simulink model "vtg_r24b"  (R2024b)
settings: Solver=FixedStepAuto  StartTime=0.0  StopTime=inf  FixedStep=0.05  RelTol=1e-3
libraries: robotlib x13
settings Model: Creator=sprinkle  LastModifiedBy=Shaimaa ElBaklish
settings OptimizationCC: DefaultParameterBehavior=Inlined  EnhancedBackFolding=on  PassReuseOutputArgsAs=Individual arguments  ZeroExternalMemoryAtStartup=off  ZeroInternalMemoryAtStartup=off  MaxStackSize=64  OptimizeBlockOrder=speed  DifferentSizesBufferReuse=on  OptimizationCustomize=off  EfficientTunableParamExpr=on
settings DebuggingCC: ParameterTunabilityLossMsg=error
settings HardwareCC: ProdBitPerPointer=32  ProdBitPerSizeT=32  ProdBitPerPtrDiffT=32  ProdLargestAtomicFloat=None  ProdIntDivRoundTo=Undefined  ProdEndianess=Unspecified  ProdWordSize=32  ProdHWDeviceType=Generic->Unspecified (assume 32-bit Generic)
settings SFSimCC: MATLABDynamicMemAlloc=off
settings RTWCC: Description=Embedded Coder  SystemTargetFile=ert.tlc  HardwareBoard=Robot Operating System (ROS)  TLCOptions="-aInlineSetEventsForThisBaseRateFcn=TLC_FALSE -aSuppressMultiTaskScheduler=TLC_FALSE  -aRateBasedStepFcn=0"  GenCodeOnly=on  TemplateMakefile=ert_default_tmf  Toolchain=Catkin  TargetLang=C++
settings CodeAppCC: ForceParamTrailComments=on  IgnoreCustomStorageClasses=off  OperatorAnnotations=on  SimulinkDataObjDesc=on  SFDataObjDesc=on  InsertBlockDesc=on

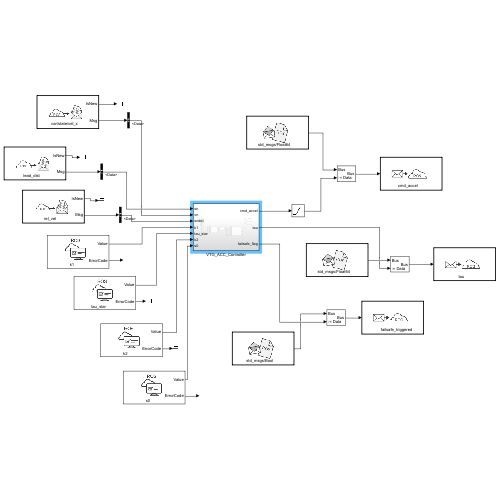
[thumbnail: Simulink's stored preview of the top-level diagram]
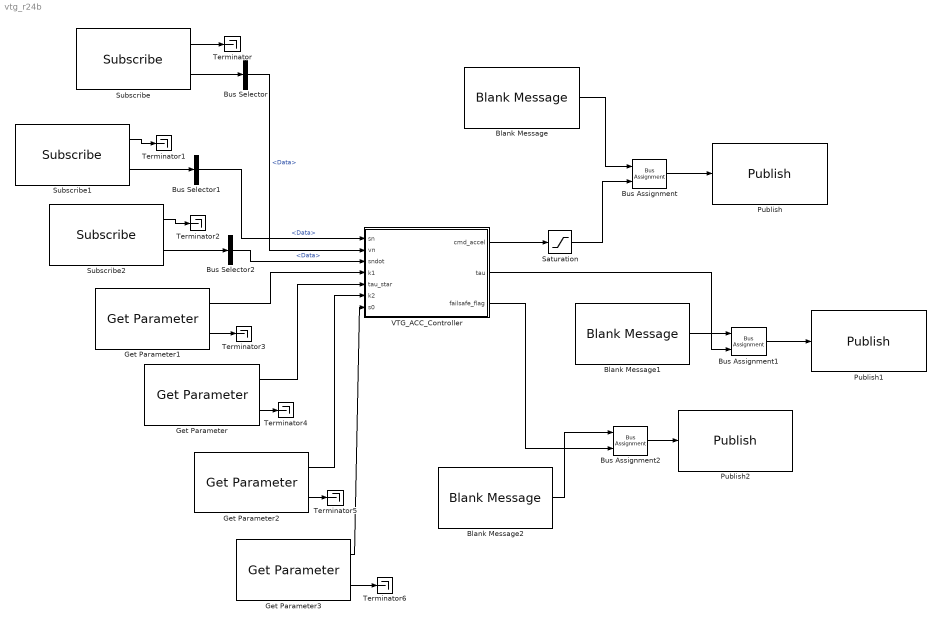
== system vtg_r24b ==
  Blank Message : robotlib/Blank Message  messageClass=Message  entityType=std_msgs/Float64  messageType=std_msgs/Float64  SampleTime=inf  legacyBusStruct=off
  Blank Message1 : robotlib/Blank Message  messageClass=Message  entityType=std_msgs/Float64  messageType=std_msgs/Float64  SampleTime=inf  legacyBusStruct=off
  Blank Message2 : robotlib/Blank Message  messageClass=Message  entityType=std_msgs/Bool  messageType=std_msgs/Bool  SampleTime=inf  legacyBusStruct=off
  Bus Assignment : BusAssignment  AssignedSignals=Data
  Bus Assignment1 : BusAssignment  AssignedSignals=Data
  Bus Assignment2 : BusAssignment  AssignedSignals=Data
  Bus Selector : BusSelector  OutputSignals=Data
  Bus Selector1 : BusSelector  OutputSignals=Data
  Bus Selector2 : BusSelector  OutputSignals=Data
  Get Parameter : robotlib/Get Parameter  ParameterSource=Specify your own  ParameterName=tau_star  ParameterType=double  ParameterMaxArrayLength=16  ParameterInitialValue=2.0  SampleTime=-1  ShowErrorCodeOutput=on  ModelName=vtg_r24b  BlockId=ParamGet_vtg_r24b_18
  Get Parameter1 : robotlib/Get Parameter  ParameterSource=Specify your own  ParameterName=k1  ParameterType=double  ParameterMaxArrayLength=16  ParameterInitialValue=1.1  SampleTime=-1  ShowErrorCodeOutput=on  ModelName=vtg_r24b  BlockId=ParamGet_vtg_r24b_19
  Get Parameter2 : robotlib/Get Parameter  ParameterSource=Specify your own  ParameterName=k2  ParameterType=double  ParameterMaxArrayLength=16  ParameterInitialValue=0.1  SampleTime=-1  ShowErrorCodeOutput=on  ModelName=vtg_r24b  BlockId=ParamGet_vtg_r24b_52
  Get Parameter3 : robotlib/Get Parameter  ParameterSource=Specify your own  ParameterName=s0  ParameterType=double  ParameterMaxArrayLength=16  ParameterInitialValue=0.1  SampleTime=-1  ShowErrorCodeOutput=on  ModelName=vtg_r24b  BlockId=ParamGet_vtg_r24b_54
  Publish : robotlib/Publish  topicSource=Specify your own  topic=cmd_accel  messageType=std_msgs/Float64  legacyBusStruct=off  messageQueueLength=1
  Publish1 : robotlib/Publish  topicSource=Specify your own  topic=tau  messageType=std_msgs/Float64  legacyBusStruct=off  messageQueueLength=1
  Publish2 : robotlib/Publish  topicSource=Specify your own  topic=failsafe_triggered  messageType=std_msgs/Float64  legacyBusStruct=off  messageQueueLength=1
  Saturation : Saturate  UpperLimit=1.5  LowerLimit=-3.0
  Subscribe : robotlib/Subscribe  topicSource=Specify your own  topic=car/state/vel_x  messageType=std_msgs/Float64  SampleTime=-1  legacyBusStruct=off  messageQueueLength=1
  Subscribe1 : robotlib/Subscribe  topicSource=Specify your own  topic=lead_dist  messageType=std_msgs/Float64  SampleTime=-1  legacyBusStruct=off  messageQueueLength=1
  Subscribe2 : robotlib/Subscribe  topicSource=Specify your own  topic=rel_vel  messageType=std_msgs/Float64  SampleTime=-1  legacyBusStruct=off  messageQueueLength=1
  Terminator{,1..6} (7 alike) : Terminator
  VTG_ACC_Controller : Subsystem
  wires:
  Subscribe/2 -> Bus Selector/1
  Subscribe/1 -> Terminator/1
  Subscribe1/1 -> Terminator1/1
  Blank Message/1 -> Bus Assignment/1
  Bus Assignment/1 -> Publish/1
  Bus Selector/1 -> VTG_ACC_Controller/2(vn)  "<Data>"
  VTG_ACC_Controller/1(cmd_accel) -> Saturation/1
  Get Parameter/1 -> VTG_ACC_Controller/5(tau_star)
  Get Parameter1/1 -> VTG_ACC_Controller/4(k1)
  Saturation/1 -> Bus Assignment/2
  Subscribe1/2 -> Bus Selector1/1
  Bus Selector1/1 -> VTG_ACC_Controller/1(sn)  "<Data>"
  Subscribe2/1 -> Terminator2/1
  Bus Selector2/1 -> VTG_ACC_Controller/3(sndot)  "<Data>"
  Subscribe2/2 -> Bus Selector2/1
  Get Parameter1/2 -> Terminator3/1
  Get Parameter/2 -> Terminator4/1
  Get Parameter2/1 -> VTG_ACC_Controller/6(k2)
  Get Parameter2/2 -> Terminator5/1
  Get Parameter3/2 -> Terminator6/1
  Get Parameter3/1 -> VTG_ACC_Controller/7(s0)
  Bus Assignment1/1 -> Publish1/1
  VTG_ACC_Controller/2(tau) -> Bus Assignment1/2
  Blank Message1/1 -> Bus Assignment1/1
  VTG_ACC_Controller/3(failsafe_flag) -> Bus Assignment2/2
  Blank Message2/1 -> Bus Assignment2/1
  Bus Assignment2/1 -> Publish2/1

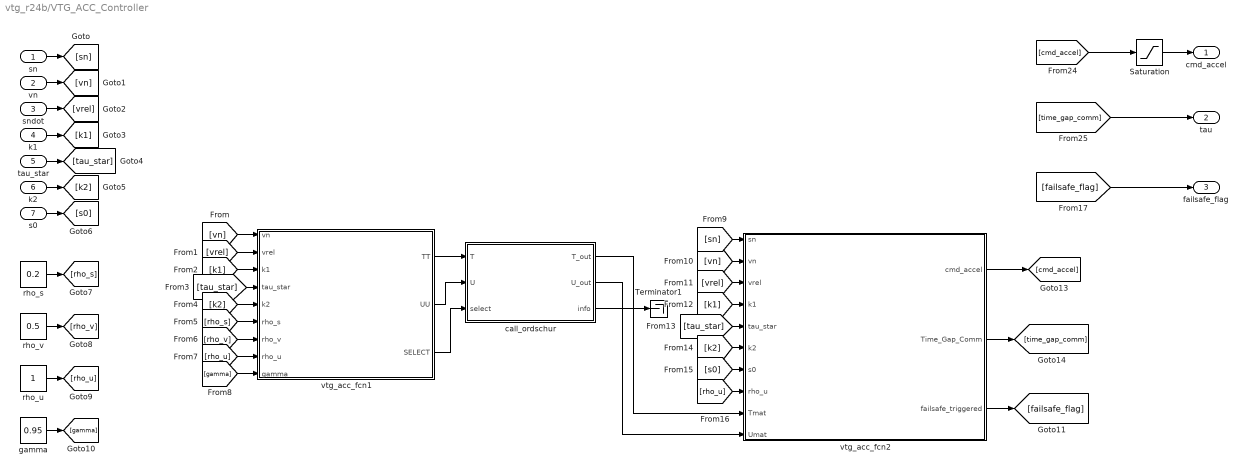
== system vtg_r24b/VTG_ACC_Controller ==
  sn : Inport
  vn : Inport  Port=2
  sndot : Inport  Port=3
  k1 : Inport  Port=4
  tau_star : Inport  Port=5
  k2 : Inport  Port=6
  s0 : Inport  Port=7
  Saturation : Saturate  UpperLimit=1.5  LowerLimit=-3
  Terminator1 : Terminator
  call_ordschur : MATLAB Function  TreatAsAtomicUnit=on
  gamma : Constant  Value=0.95
  rho_s : Constant  Value=0.2
  rho_u : Constant
  rho_v : Constant  Value=0.5
  vtg_acc_fcn1 : MATLAB Function  TreatAsAtomicUnit=on
  vtg_acc_fcn2 : MATLAB Function  TreatAsAtomicUnit=on
  cmd_accel : Outport
  tau : Outport  Port=2
  failsafe_flag : Outport  Port=3
  wires:
  Saturation/1 -> cmd_accel/1
  vtg_acc_fcn1/1(TT) -> call_ordschur/1(T)
  vtg_acc_fcn1/2(UU) -> call_ordschur/2(U)
  vtg_acc_fcn1/3(SELECT) -> call_ordschur/3(select)
  call_ordschur/1(T_out) -> vtg_acc_fcn2/9(Tmat)
  call_ordschur/3(info) -> Terminator1/1
  sn/1 -> [sn]
  vn/1 -> [vn]
  sndot/1 -> [vrel]
  k1/1 -> [k1]
  tau_star/1 -> [tau_star]
  k2/1 -> [k2]
  s0/1 -> [s0]
  rho_s/1 -> [rho_s]
  rho_v/1 -> [rho_v]
  rho_u/1 -> [rho_u]
  gamma/1 -> [gamma]
  [vn] -> vtg_acc_fcn1/1(vn)
  [vrel] -> vtg_acc_fcn1/2(vrel)
  [k1] -> vtg_acc_fcn1/3(k1)
  [tau_star] -> vtg_acc_fcn1/4(tau_star)
  [k2] -> vtg_acc_fcn1/5(k2)
  [rho_s] -> vtg_acc_fcn1/6(rho_s)
  [rho_v] -> vtg_acc_fcn1/7(rho_v)
  [rho_u] -> vtg_acc_fcn1/8(rho_u)
  [gamma] -> vtg_acc_fcn1/9(gamma)
  [sn] -> vtg_acc_fcn2/1(sn)
  [vn] -> vtg_acc_fcn2/2(vn)
  [vrel] -> vtg_acc_fcn2/3(vrel)
  [k1] -> vtg_acc_fcn2/4(k1)
  [tau_star] -> vtg_acc_fcn2/5(tau_star)
  [k2] -> vtg_acc_fcn2/6(k2)
  [s0] -> vtg_acc_fcn2/7(s0)
  [rho_u] -> vtg_acc_fcn2/8(rho_u)
  [cmd_accel] -> Saturation/1
  [time_gap_comm] -> tau/1
  vtg_acc_fcn2/1(cmd_accel) -> [cmd_accel]
  vtg_acc_fcn2/2(Time_Gap_Comm) -> [time_gap_comm]
  vtg_acc_fcn2/3(failsafe_triggered) -> [failsafe_flag]
  [failsafe_flag] -> failsafe_flag/1
  call_ordschur/2(U_out) -> vtg_acc_fcn2/10(Umat)

== matlab function vtg_r24b/VTG_ACC_Controller/vtg_acc_fcn1 ==
  data: TT output; vn input; vrel input; k1 input; tau_star input; k2 input; UU output; rho_s input; rho_v input; rho_u input; gamma input; SELECT output
function [TT, UU, SELECT] = vtg_acc_fcn1(vn, vrel, k1, tau_star, k2, rho_s, rho_v, rho_u, gamma)
Asys = [0 -1; k1 (-k1*tau_star-k2)];
Bdist = [1; k2];
Csys = [rho_s 0; 0 rho_v; 0 0];
Ru = rho_u^2;
Rmat = [-1/gamma^2 0; 0 inv(Ru)];

ve = vrel + vn;
Bctrl = [0; -k1*ve];

Bsys = [Bdist, Bctrl];
Qmat = Csys'*Csys;

% --- Replacement for icare(A, B, Q, R) -----------------------------------
Z = [Asys -(Bsys/Rmat*Bsys'); -Qmat -Asys']; % Hamiltonian
[UU, TT] = schur(Z);
SELECT0 = real(ordeig(TT)) < 0;
SELECT0 = logical(SELECT0);
SELECT = int32(SELECT0);  % Already length 4, no expansion
end

== matlab function vtg_r24b/VTG_ACC_Controller/call_ordschur ==
  data: T input; T_out output; U input; select input; U_out output; info output
function [T_out, U_out, info] = call_ordschur(T, U, select)
%#codegen
coder.cinclude('ordschur_wrapper.h');

n = size(T,1);

T_out = T;
U_out = U;

info = int32(0);

info = coder.ceval('ordschur_reorder', ...
    int32(n), ...
    coder.ref(T_out), ...
    coder.ref(U_out), ...
    coder.rref(select) );

% For Simulink
customDir = "C:\Users\ShaimaaElBaklish\Documents\GitHub\vtg_acc_real\simulink\mycfiles";
coder.updateBuildInfo('addIncludePaths', customDir);
coder.updateBuildInfo('addSourcePaths', customDir);
coder.updateBuildInfo('addSourceFiles', 'ordschur_wrapper.c');
end

== matlab function vtg_r24b/VTG_ACC_Controller/vtg_acc_fcn2 ==
  data: sn input; cmd_accel output; vn input; vrel input; k1 input; tau_star input; k2 input; s0 input; rho_u input; Time_Gap_Comm output; Tmat input; failsafe_triggered output; Umat input
function [cmd_accel, Time_Gap_Comm, failsafe_triggered] = vtg_acc_fcn2(sn, vn, vrel, k1, tau_star, k2, s0, rho_u, Tmat, Umat)
cmd_accel = 0; Time_Gap_Comm= 0; failsafe_triggered = false;
Ru = rho_u^2;

ve = vrel + vn;
s_err = sn - (s0+tau_star*ve);
v_err = vn - ve;

% --- Replacement for icare(A, B, Q, R) -----------------------------------
P = zeros(2, 2);
[m,n] = size(Umat);
U11 = Umat(1:(m/2), 1:(n/2));
U21 = Umat((m/2+1):m, 1:(n/2));
P = U21/U11;
% -------------------------------------------------------------------------

ui = -inv(Ru)*([0 -k1*vn]*P*[s_err; v_err]);

% ── Check failsafe condition ───────────────────────────────────
diagT = diag(Tmat);
n     = length(diagT)/2;
failsafe_triggered = ~(all(diagT(1:n) < 0) && all(diagT(n+1:end) > 0));
if failsafe_triggered
    Time_Gap_Comm = tau_star;
else
    Time_Gap_Comm = max(tau_star + double(ui), 0);
end

cmd_accel = k1*(sn-s0-Time_Gap_Comm*vn) + k2*vrel;
end
